simulink model "microgrid_simulation"  (R2023b)
settings: Solver=FixedStepAuto  StartTime=0.0  StopTime=288  FixedStep=1  RelTol=1e-3
libraries: simulink x1
settings Model: Creator=nilki  LastModifiedBy=nilki

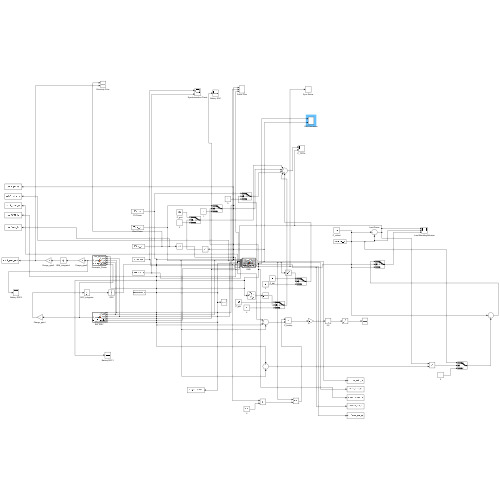
[thumbnail: Simulink's stored preview of the top-level diagram]
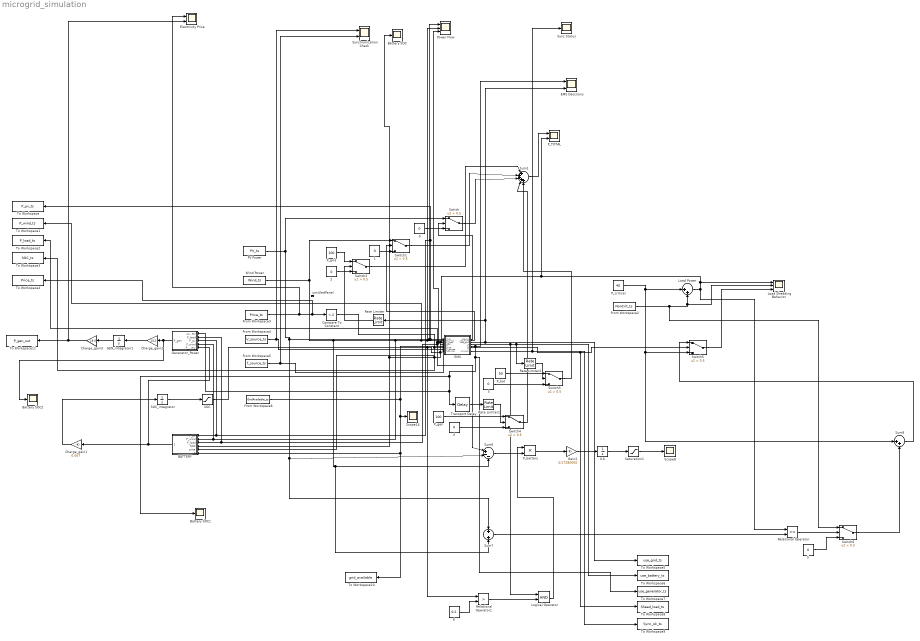
== system microgrid_simulation ==
  {0..5} (6 alike) : Constant  Value=0
  0.6 : Integrator  InitialCondition=0.6
  6 : Constant  Value=0.2
  BATTERY : MATLAB Function  TreatAsAtomicUnit=on
  Battery SOC : Scope
  Battery SOC1 : Scope
  Battery SOC2 : Scope
  Charge_gain1 : Gain  Gain=0.007
  Charge_gain2 : Gain  Gain=1/12
  Charge_gain3 : Gain  Gain=19.5
  Compare To Constant : simulink/Logic and Bit Operations/Compare To Constant  relop=<  const=2  OutDataTypeStr=boolean
  EMS : MATLAB Function  TreatAsAtomicUnit=on
  EMS Decisions : Scope  NumInputPorts=2
  Electricity Price : Scope  NumInputPorts=2
  From Workspace2 : FromWorkspace  VariableName=NonCrit_ts  SampleTime=-1
  From Workspace3 : FromWorkspace  VariableName=Price_ts  SampleTime=-1
  From Workspace4 : FromWorkspace  VariableName=V_source_ts  SampleTime=-1
  From Workspace5 : FromWorkspace  VariableName=f_source_ts  SampleTime=-1
  From Workspace6 : FromWorkspace  VariableName=GridAvailable_ts  SampleTime=-1
  GEN_integrator1 : Integrator
  Gain2 : Gain  Gain=-1/17280000
  Generator_Power : MATLAB Function  TreatAsAtomicUnit=on
  Load Power : Sum  Inputs=|++
  Load Shedding Behavior : Scope  NumInputPorts=3
  Logical Operator : Logic  AllPortsSameDT=off  OutDataTypeStr=boolean
  PV Power : FromWorkspace  VariableName=PV_ts  SampleTime=-1
  P_TOTAL : Scope  NumInputPorts=2
  P_bat : Constant  Value=50
  P_battery : Product
  P_critical : Constant  Value=40
  P_gen : Constant  Value=100
  P_grid : Constant  Value=100
  Power Flow : Scope  NumInputPorts=3
  Rate Limiter : RateLimiter  RisingSlewLimit=0.5  FallingSlewLimit=-0.5  SampleTimeMode=inherited
  Rate Limiter1 : RateLimiter  RisingSlewLimit=0.5  FallingSlewLimit=-0.5  SampleTimeMode=inherited
  Rate Limiter2 : RateLimiter  RisingSlewLimit=0.5  FallingSlewLimit=-0.5  SampleTimeMode=inherited
  Relational Operator : RelationalOperator  OutDataTypeStr=boolean  RndMeth=Simplest  InputSameDT=off
  Relational Operator1 : RelationalOperator  Operator=>  OutDataTypeStr=boolean  RndMeth=Simplest  InputSameDT=off
  SOC : Saturate  UpperLimit=0.9  LowerLimit=0.2
  SOC_integrator : Integrator  InitialCondition=0.6
  Saturation1 : Saturate  UpperLimit=1  LowerLimit=0
  Scope14 : Scope
  Scope8 : Scope
  Sum1 : Sum  Inputs=|+++++
  Sum6 : Sum  Inputs=|+--
  Sum7 : Sum
  Sum8 : Sum  Inputs=|++
  Switch{,1..6} (7 alike) : Switch  Criteria=u2 > Threshold  Threshold=0.5  SaturateOnIntegerOverflow=off  InputSameDT=off
  Sync Status : Scope
  Synchronization Check : Scope  NumInputPorts=2
  To Workspace : ToWorkspace  VariableName=P_pv_ts  SaveFormat=Timeseries  SampleTime=-1
  To Workspace1 : ToWorkspace  VariableName=P_wind_ts  SaveFormat=Timeseries  SampleTime=-1
  To Workspace10 : ToWorkspace  VariableName=grid_available  SaveFormat=Timeseries  SampleTime=-1
  To Workspace11 : ToWorkspace  VariableName=P_gen_out  SampleTime=-1
  To Workspace2 : ToWorkspace  VariableName=P_load_ts  SaveFormat=Timeseries  SampleTime=-1
  To Workspace3 : ToWorkspace  VariableName=SOC_ts  SaveFormat=Timeseries  SampleTime=-1
  To Workspace4 : ToWorkspace  VariableName=Price_ts  SaveFormat=Timeseries  SampleTime=-1
  To Workspace5 : ToWorkspace  VariableName=use_grid_ts  SaveFormat=Timeseries  SampleTime=-1
  To Workspace6 : ToWorkspace  VariableName=use_battery_ts  SaveFormat=Timeseries  SampleTime=-1
  To Workspace7 : ToWorkspace  VariableName=use_generator_ts  SaveFormat=Timeseries  SampleTime=-1
  To Workspace8 : ToWorkspace  VariableName=Shead_load_ts  SaveFormat=Timeseries  SampleTime=-1
  To Workspace9 : ToWorkspace  VariableName=Sync_ok_ts  SaveFormat=Timeseries  SampleTime=-1
  Transport Delay : TransportDelay  DelayTime=2
  Wind Power : FromWorkspace  VariableName=Wind_ts  SampleTime=-1
  untitledPanel : Subsystem  Tag=HiddenForWebPanel  IsWebBlockPanel=on
  wires:
  EMS/2(use_wind) -> Switch1/2
  From Workspace6/1 -> To Workspace10/1, BATTERY/6(grid_available), Scope14/1, EMS/5(grid_available)
  EMS/1(use_pv) -> Switch/2
  EMS/3(use_grid) -> To Workspace5/1, EMS Decisions/2, Rate Limiter/1
  0/1 -> Switch/3
  1/1 -> Switch1/3
  2/1 -> Switch2/3
  PV Power/1 -> Switch/1, Sum7/1, Sum6/2, Power Flow/1, To Workspace/1, Generator_Power/3(P_pv), BATTERY/1(P_pv), EMS/1(P_pv)
  Wind Power/1 -> Switch1/1, Sum7/2, Sum6/3, To Workspace1/1, Power Flow/2, EMS/2(P_wind), Generator_Power/4(P_wind), BATTERY/2(P_wind)
  P_grid/1 -> Switch2/1
  Switch2/1 -> Sum1/1
  Switch1/1 -> Sum1/2
  Switch/1 -> Sum1/3
  Sum1/1 -> P_TOTAL/1
  3/1 -> Switch3/3
  EMS/4(use_battery) -> Logical Operator/1, To Workspace6/1, Rate Limiter2/1
  P_gen/1 -> Switch4/1
  4/1 -> Switch4/3
  EMS/5(use_generator) -> EMS Decisions/1, To Workspace7/1, Battery SOC1/1, Generator_Power/1(use_generator), Transport Delay/1
  Switch4/1 -> Sum1/4
  Switch3/1 -> Sum1/5
  P_critical/1 -> Load Power/1, Sum8/1, Switch5/3
  EMS/6(shed_load) -> To Workspace8/1, Switch5/2
  SOC_integrator/1 -> SOC/1
  Sum6/1 -> P_battery/2
  P_battery/1 -> Gain2/1
  Gain2/1 -> 0.6/1
  0.6/1 -> Saturation1/1
  Saturation1/1 -> Scope8/1
  Sum7/1 -> Relational Operator/2
  Relational Operator/1 -> Switch6/2
  5/1 -> Switch6/3
  Switch6/1 -> Sum8/2
  Sum8/1 -> Switch5/1
  6/1 -> Relational Operator1/2
  Relational Operator1/1 -> Logical Operator/2
  Logical Operator/1 -> P_battery/1
  SOC/1 -> Relational Operator1/1, BATTERY/4(SOC), Battery SOC/1, To Workspace3/1, EMS/4(SOC)
  Load Power/1 -> Load Shedding Behavior/1, P_TOTAL/2, Power Flow/3, Generator_Power/2(P_load), BATTERY/3(P_load), Sum6/1, To Workspace2/1, EMS/3(P_load), Relational Operator/1
  From Workspace2/1 -> Switch6/1, Load Shedding Behavior/2, Load Power/2
  P_bat/1 -> Switch3/1
  From Workspace4/1 -> Synchronization Check/1, EMS/7(V_source)
  From Workspace5/1 -> Synchronization Check/2, EMS/8(f_source)
  Rate Limiter/1 -> Switch2/2
  Transport Delay/1 -> Rate Limiter1/1
  Rate Limiter1/1 -> Switch4/2
  Rate Limiter2/1 -> Switch3/2
  From Workspace3/1 -> Electricity Price/1, To Workspace4/1, Compare To Constant/1
  Switch5/1 -> Load Shedding Behavior/3
  EMS/8(sync_ok) -> To Workspace9/1, Sync Status/1
  Compare To Constant/1 -> EMS/6(price), BATTERY/5(price)
  Charge_gain1/1 -> SOC_integrator/1
  BATTERY/1(P_battery) -> Charge_gain1/1, Generator_Power/5(P_battery)
  Charge_gain2/1 -> GEN_integrator1/1
  GEN_integrator1/1 -> Charge_gain3/1
  Generator_Power/1(P_gen) -> Battery SOC2/1, Charge_gain2/1
  Charge_gain3/1 -> Electricity Price/2, To Workspace11/1

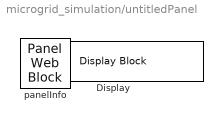
== system microgrid_simulation/untitledPanel ==
  Display : DisplayBlock  Tag=HiddenForWebPanel  PanelInfo="{\"addnFilesFolder\":\"\",\"height\":40,\"includeDebugPackages\":false,\"left\":18,\"outputFolder\":\"\",\"panelId\":\"panelId-82cdfdf6-3aee-4c5e-86f1-598b490c3b8d\",\"popoutMode\":\"\",\"standaloneTitle\":\"\",\"top\":18,\"type\":\"panelChild\",\"version\":\"2019b\",\"width\":180,\"zIndex\":1500002}"  LabelPosition=Hide  Transparency=1
  panelInfo : PanelWebBlock  Tag=HiddenForWebPanel  PanelInfo="{\"addnFilesFolder\":\"\",\"compacted\":false,\"height\":80,\"includeDebugPackages\":false,\"isActiveTab\":true,\"left\":41,\"name\":\"Panel\",\"outputFolder\":\"\",\"panelId\":\"panelId-82cdfdf6-3aee-4c5e-86f1-598b490c3b8d\",\"popoutMode\":\"\",\"standaloneTitle\":\"\",\"tabIndex\":0,\"tabbedSetId\":\"tabbedSet8026185298\",\"top\":575,\"type\":\"panel\",\"version\":\"2019b\",\"visible\":true,\"width\":220,\"zIndex\":1500002}"

== matlab function microgrid_simulation/BATTERY ==
  data: P_pv input; P_battery output; P_wind input; P_load input; SOC input; price input; grid_available input
function P_battery = Battery_Power_Control(P_pv, P_wind, P_load, SOC, price, grid_available)

% =========================
% PARAMETRELER
% =========================
SOC_min = 0.20;
SOC_max = 0.90;

price_low = 1.50;

P_charge_max = 40;       % kW - fazla yenilenebilir şarj
P_discharge_max = 40;    % kW - batarya deşarj
P_grid_charge = 15;      % kW - gece/ucuz şebeke şarjı

% =========================
% GÜÇ HESAPLARI
% =========================
P_renew = P_pv + P_wind;
P_fark = P_renew - P_load;

P_battery = 0;

% P_battery > 0  : batarya şarj oluyor
% P_battery < 0  : batarya deşarj oluyor

% =========================
% 1) Fazla yenilenebilir varsa batarya dolar
% =========================
if P_fark > 0 && SOC < SOC_max

    P_battery = min(P_fark, P_charge_max);

% =========================
% 2) Yenilenebilir yetmiyor ama gece/ucuz şebeke varsa
% Eksik güç şebekeden karşılanır, batarya da şarj olur
% =========================
elseif P_fark <= 0 && grid_available == 1 && price <= price_low && SOC < SOC_max

    P_battery = P_grid_charge;

% =========================
% 3) Ucuz şebeke yoksa batarya eksik gücü tamamlar
% =========================
elseif P_fark < 0 && SOC > SOC_min

    P_battery = -min(-P_fark, P_discharge_max);

% =========================
% 4) Diğer durumlarda batarya pasif
% =========================
else

    P_battery = 0;

end

end

== matlab function microgrid_simulation/EMS ==
  data: P_pv input; use_pv output; P_wind input; P_load input; SOC input; grid_available input; use_wind output; use_grid output; use_battery output; use_generator output; shed_load output; charge_battery output; price input; V_source input; f_source input; sync_ok output
function [use_pv, use_wind, use_grid, use_battery, use_generator, shed_load, charge_battery, sync_ok] = ...
    EMS_Control(P_pv, P_wind, P_load, SOC, grid_available, price, V_source, f_source)

% =========================
% PARAMETRELER
% =========================
SOC_min = 0.20;
SOC_max = 0.85;

price_low = 1.50;

V_ref = 400;
f_ref = 50;

V_tol = 0.02;
f_tol = 0.10;

% =========================
% BAŞLANGIÇ
% =========================
use_pv = 0;
use_wind = 0;
use_grid = 0;
use_battery = 0;
use_generator = 0;
shed_load = 0;
charge_battery = 0;
sync_ok = 0;

% =========================
% SENKRON KONTROL
% =========================
V_min = V_ref * (1 - V_tol);
V_max = V_ref * (1 + V_tol);

f_min = f_ref - f_tol;
f_max = f_ref + f_tol;

if grid_available == 1 && ...
   V_source >= V_min && V_source <= V_max && ...
   f_source >= f_min && f_source <= f_max
    sync_ok = 1;
end

% =========================
% YENİLENEBİLİR KAYNAKLAR
% =========================
if P_pv > 0
    use_pv = 1;
end

if P_wind > 0
    use_wind = 1;
end

P_renewable = P_pv + P_wind;
deficit = P_load - P_renewable;

% =========================
% EMS KARAR MANTIĞI
% =========================

% 1) Yenilenebilir üretim yükü karşılıyorsa
if deficit <= 0

    use_grid = 0;
    use_battery = 0;
    use_generator = 0;
    shed_load = 0;

    % Fazla yenilenebilir varsa batarya şarj
    if SOC < SOC_max
        charge_battery = 1;
    end

% 2) Yenilenebilir üretim yükü karşılamıyorsa
else

    % 2A) Gece/ucuz şebeke varsa:
    % Eksik güç şebekeden karşılanır, batarya da şarj edilir
    if sync_ok == 1 && price <= price_low && SOC < SOC_max

        use_grid = 1;
        charge_battery = 1;
        use_battery = 0;
        use_generator = 0;
        shed_load = 0;

    % 2B) Ucuz değilse ve batarya yeterliyse:
    % Eksik güç bataryadan karşılanır
    elseif SOC > SOC_min

        use_battery = 1;
        use_grid = 0;
        charge_battery = 0;
        use_generator = 0;
        shed_load = 0;

    % 2C) Batarya düşükse ve şebeke uygunsa:
    % Eksik güç şebekeden karşılanır
    elseif sync_ok == 1

        use_grid = 1;
        use_battery = 0;
        charge_battery = 0;
        use_generator = 0;
        shed_load = 0;

    % 2D) Şebeke yok ve batarya düşükse:
    % Jeneratör + kritik olmayan yük atma
    else

        use_grid = 0;
        use_battery = 0;
        charge_battery = 0;
        use_generator = 1;
        shed_load = 1;

    end
end

% =========================
% GÜVENLİK
% =========================
if charge_battery == 1
    use_battery = 0;
end

if use_grid == 1
    use_generator = 0;
    shed_load = 0;
end

end

== matlab function microgrid_simulation/Generator_Power ==
  data: use_generator input; P_load input; P_pv input; P_gen output; P_wind input; P_battery input
function P_gen = Generator_Power(use_generator, P_load, P_pv, P_wind, P_battery)

remaining_power = max(0, P_load - (P_pv + P_wind + P_battery));

if use_generator == 1

    P_gen = min(100, remaining_power);

else

    P_gen = 0;

end
